simulink model "statespaceexamples"  (R2013b)
settings: Solver=ode45  StartTime=0.0  StopTime=1  MaxStep=1e-3  RelTol=1e-3
settings Model: Creator=r.sipahi  LastModifiedBy=r.sipahi

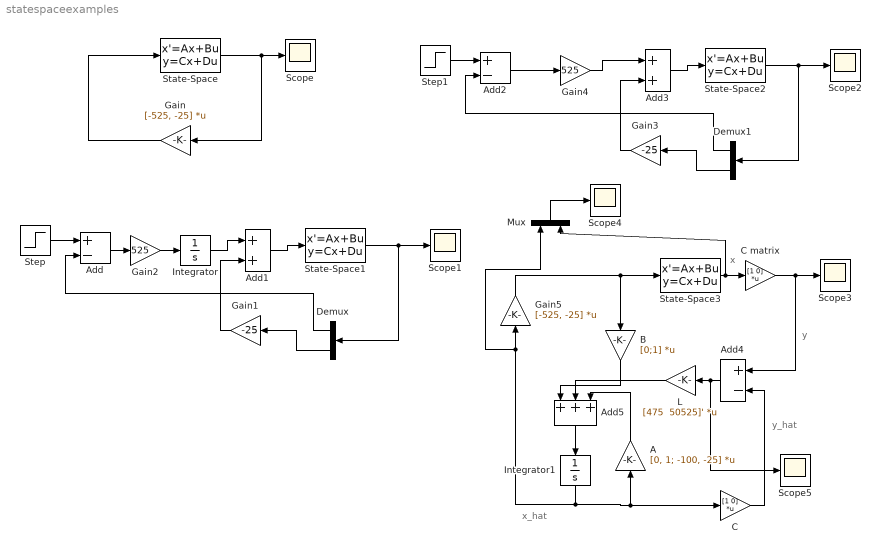
== system statespaceexamples ==
  note: x_hat
  note: x
  note: y_hat
  note: y
  A : Gain  Gain=[0, 1; -100, -25]  Multiplication=Matrix(K*u)
  Add : Sum  Inputs=+-
  Add1 : Sum
  Add2 : Sum  Inputs=+-
  Add3 : Sum
  Add4 : Sum  Inputs=+-
  Add5 : Sum  Inputs=+++
  B : Gain  Gain=[0;1]  Multiplication=Matrix(K*u)
  C : Gain  Gain=[1 0]  Multiplication=Matrix(K*u)
  C matrix : Gain  Gain=[1 0]  Multiplication=Matrix(K*u)
  Demux : Demux  Outputs=2
  Demux1 : Demux  Outputs=2
  Gain : Gain  Gain=[-525, -25]  Multiplication=Matrix(K*u)
  Gain1 : Gain  Gain=-25
  Gain2 : Gain  Gain=525
  Gain3 : Gain  Gain=-25
  Gain4 : Gain  Gain=525
  Gain5 : Gain  Gain=[-525, -25]  Multiplication=Matrix(K*u)
  Integrator : Integrator
  Integrator1 : Integrator
  L : Gain  Gain="[475  50525]'"  Multiplication=Matrix(K*u)
  Mux : Mux  Inputs=2
  Scope{,1..5} (6 alike) : Scope
      Scope2 settings: SaveName=ScopeData2
      Scope3 settings: SaveName=ScopeData3
      Scope4 settings: SaveName=ScopeData4
      Scope5 settings: SaveName=ScopeData5
  State-Space : StateSpace  A=[0, 1; -100, -25]  B=[0;1]  C=eye(2)  D=[0;0]  X0=[1;0]
  State-Space1 : StateSpace  A=[0, 1; -100, -25]  B=[0;1]  C=eye(2)  D=[0;0]  X0=[1;0]
  State-Space2 : StateSpace  A=[0, 1; -100, -25]  B=[0;1]  C=eye(2)  D=[0;0]  X0=[1;0]
  State-Space3 : StateSpace  A=[0, 1; -100, -25]  B=[0;1]  C=eye(2)  D=[0; 0]  X0=[1;0]
  Step : Step  Time=0  SampleTime=0
  Step1 : Step  Time=0  SampleTime=0
  wires:
  State-Space/1 -> Scope/1, Gain/1
  Gain/1 -> State-Space/1
  State-Space1/1 -> Demux/1, Scope1/1
  Step/1 -> Add/1
  Add/1 -> Gain2/1
  Gain2/1 -> Integrator/1
  Gain1/1 -> Add1/2
  Add1/1 -> State-Space1/1
  Demux/2 -> Gain1/1
  Demux/1 -> Add/2
  Integrator/1 -> Add1/1
  State-Space2/1 -> Scope2/1, Demux1/1
  Step1/1 -> Add2/1
  Add2/1 -> Gain4/1
  Gain3/1 -> Add3/2
  Add3/1 -> State-Space2/1
  Demux1/2 -> Gain3/1
  Demux1/1 -> Add2/2
  Gain4/1 -> Add3/1
  State-Space3/1 -> Mux/2, C matrix/1
  Gain5/1 -> State-Space3/1, B/1
  Integrator1/1 -> C/1, A/1, Mux/1, Gain5/1
  C/1 -> Add4/2
  Add4/1 -> Scope5/1, L/1
  B/1 -> Add5/1
  L/1 -> Add5/2
  A/1 -> Add5/3
  Add5/1 -> Integrator1/1
  C matrix/1 -> Add4/1, Scope3/1
  Mux/1 -> Scope4/1
